simulink model "TST_Fan_DD"  (R2016b)
settings: Solver=FixedStepDiscrete  StartTime=0.0  StopTime=simTime  FixedStep=sampleTime  RelTol=1e-3
values from neighbouring files (symbols this model uses):
  testCase = 1    [initTST_Fan_DD_001.m]    (also in initTST_Fan_DD_002.m = 2)
libraries: simulink x13, UnitTest_Lib x10
settings Model: Creator=liangyunbo  LastModifiedBy=liangyunbo
settings DebuggingCC: SignalRangeChecking=error

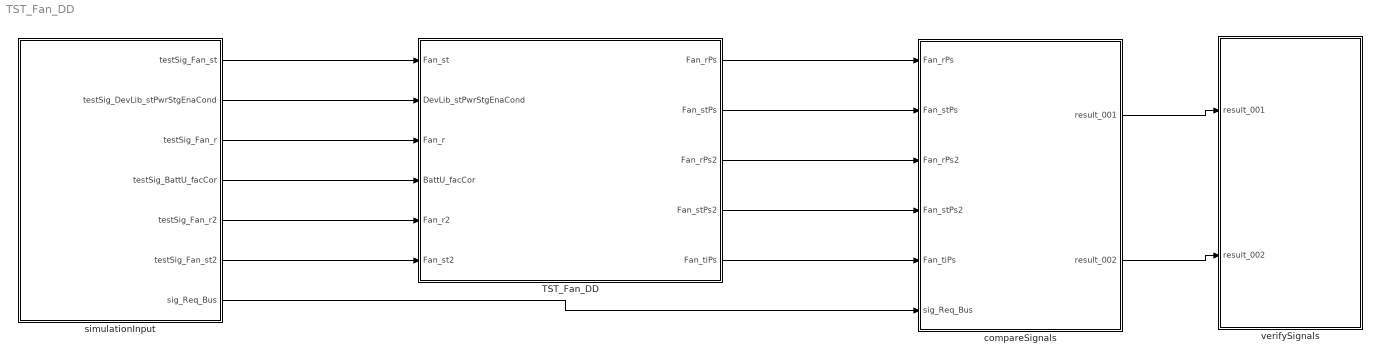
== system TST_Fan_DD ==
  TST_Fan_DD : Subsystem
  compareSignals : Subsystem
  simulationInput : Subsystem
  verifySignals : Subsystem
  wires:
  simulationInput/1(testSig_Fan_st) -> TST_Fan_DD/1(Fan_st)
  simulationInput/2(testSig_DevLib_stPwrStgEnaCond) -> TST_Fan_DD/2(DevLib_stPwrStgEnaCond)
  simulationInput/3(testSig_Fan_r) -> TST_Fan_DD/3(Fan_r)
  simulationInput/4(testSig_BattU_facCor) -> TST_Fan_DD/4(BattU_facCor)
  simulationInput/5(testSig_Fan_r2) -> TST_Fan_DD/5(Fan_r2)
  simulationInput/6(testSig_Fan_st2) -> TST_Fan_DD/6(Fan_st2)
  TST_Fan_DD/1(Fan_rPs) -> compareSignals/1(Fan_rPs)
  TST_Fan_DD/2(Fan_stPs) -> compareSignals/2(Fan_stPs)
  TST_Fan_DD/3(Fan_rPs2) -> compareSignals/3(Fan_rPs2)
  TST_Fan_DD/4(Fan_stPs2) -> compareSignals/4(Fan_stPs2)
  TST_Fan_DD/5(Fan_tiPs) -> compareSignals/5(Fan_tiPs)
  simulationInput/7(sig_Req_Bus) -> compareSignals/6(sig_Req_Bus)
  compareSignals/1(result_001) -> verifySignals/1(result_001)
  compareSignals/2(result_002) -> verifySignals/2(result_002)

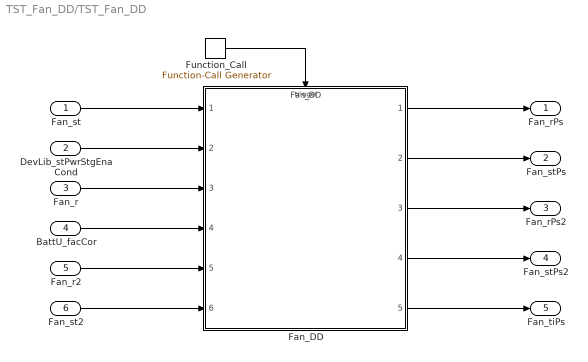
== system TST_Fan_DD/TST_Fan_DD ==
  Fan_st : Inport
  DevLib_stPwrStgEnaCond : Inport  Port=2
  Fan_r : Inport  Port=3
  BattU_facCor : Inport  Port=4
  Fan_r2 : Inport  Port=5
  Fan_st2 : Inport  Port=6
  Fan_DD : ModelReference  ModelNameDialog=Fan_DD  SimulationMode=Normal  ModelReferenceVersion=1.95  TriggerPortName=function  TriggerPortTriggerType=function-call  TriggerPortStatesWhenEnabling=held
  Function_Call : simulink/Ports & Subsystems/Function-Call Generator  sample_time=sampleTime  numberOfIterations=1
  Fan_rPs : Outport
  Fan_stPs : Outport  Port=2
  Fan_rPs2 : Outport  Port=3
  Fan_stPs2 : Outport  Port=4
  Fan_tiPs : Outport  Port=5
  wires:
  Function_Call/1 -> Fan_DD/Trigger
  Fan_st/1 -> Fan_DD/1
  DevLib_stPwrStgEnaCond/1 -> Fan_DD/2
  Fan_r/1 -> Fan_DD/3
  BattU_facCor/1 -> Fan_DD/4
  Fan_r2/1 -> Fan_DD/5
  Fan_st2/1 -> Fan_DD/6
  Fan_DD/1 -> Fan_rPs/1
  Fan_DD/2 -> Fan_stPs/1
  Fan_DD/3 -> Fan_rPs2/1
  Fan_DD/4 -> Fan_stPs2/1
  Fan_DD/5 -> Fan_tiPs/1

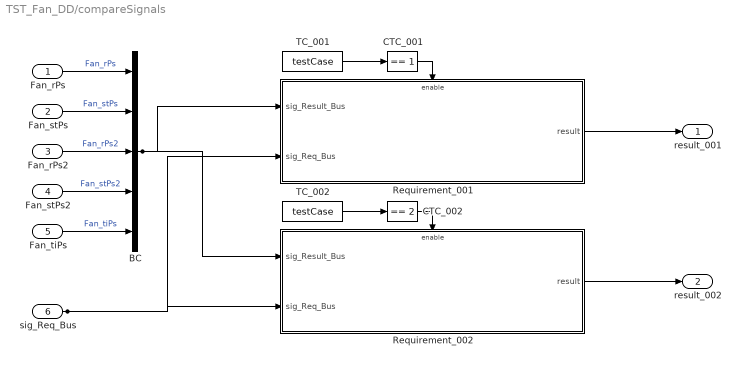
== system TST_Fan_DD/compareSignals ==
  Fan_rPs : Inport
  Fan_stPs : Inport  Port=2
  Fan_rPs2 : Inport  Port=3
  Fan_stPs2 : Inport  Port=4
  Fan_tiPs : Inport  Port=5
  sig_Req_Bus : Inport  Port=6
  BC : BusCreator  Inputs=5
  CTC_001 : simulink/Logic and Bit Operations/Compare To Constant  relop===  const=1  OutDataTypeStr=boolean
  CTC_002 : simulink/Logic and Bit Operations/Compare To Constant  relop===  const=2  OutDataTypeStr=boolean
  Requirement_001 : Subsystem
  Requirement_002 : Subsystem
  TC_001 : Constant  Value=testCase
  TC_002 : Constant  Value=testCase
  result_001 : Outport
  result_002 : Outport  Port=2
  wires:
  Fan_rPs/1 -> BC/1  "Fan_rPs"
  Fan_stPs/1 -> BC/2  "Fan_stPs"
  Fan_rPs2/1 -> BC/3  "Fan_rPs2"
  Fan_stPs2/1 -> BC/4  "Fan_stPs2"
  Fan_tiPs/1 -> BC/5  "Fan_tiPs"
  TC_001/1 -> CTC_001/1
  CTC_001/1 -> Requirement_001/Enable
  sig_Req_Bus/1 -> Requirement_001/2(sig_Req_Bus), Requirement_002/2(sig_Req_Bus)
  BC/1 -> Requirement_001/1(sig_Result_Bus), Requirement_002/1(sig_Result_Bus)
  Requirement_001/1(result) -> result_001/1
  TC_002/1 -> CTC_002/1
  CTC_002/1 -> Requirement_002/Enable
  Requirement_002/1(result) -> result_002/1

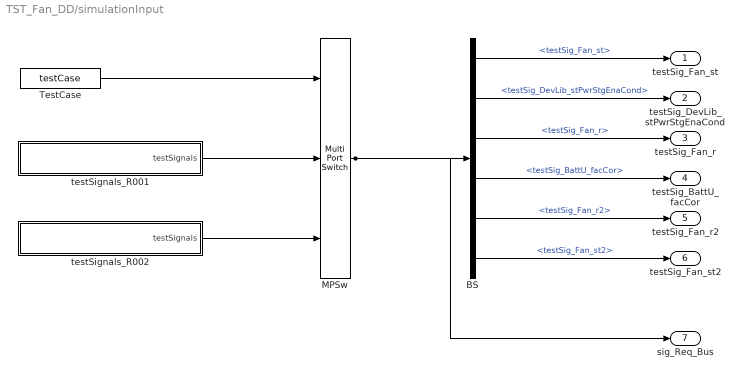
== system TST_Fan_DD/simulationInput ==
  BS : BusSelector  OutputSignals=testSig_Fan_st,testSig_DevLib_stPwrStgEnaCond,testSig_Fan_r,testSig_BattU_facCor,testSig_Fan_r2,testSig_Fan_st2
  MPSw : MultiPortSwitch  Inputs=2  SaturateOnIntegerOverflow=on  InputSameDT=on
  TestCase : Constant  Value=testCase
  testSignals_R001 : Subsystem
  testSignals_R002 : Subsystem
  testSig_Fan_st : Outport
  testSig_DevLib_stPwrStgEnaCond : Outport  Port=2
  testSig_Fan_r : Outport  Port=3
  testSig_BattU_facCor : Outport  Port=4
  testSig_Fan_r2 : Outport  Port=5
  testSig_Fan_st2 : Outport  Port=6
  sig_Req_Bus : Outport  Port=7
  wires:
  BS/1 -> testSig_Fan_st/1  "<testSig_Fan_st>"
  BS/2 -> testSig_DevLib_stPwrStgEnaCond/1  "<testSig_DevLib_stPwrStgEnaCond>"
  BS/3 -> testSig_Fan_r/1  "<testSig_Fan_r>"
  BS/4 -> testSig_BattU_facCor/1  "<testSig_BattU_facCor>"
  BS/5 -> testSig_Fan_r2/1  "<testSig_Fan_r2>"
  BS/6 -> testSig_Fan_st2/1  "<testSig_Fan_st2>"
  MPSw/1 -> BS/1, sig_Req_Bus/1
  TestCase/1 -> MPSw/1
  testSignals_R001/1(testSignals) -> MPSw/2
  testSignals_R002/1(testSignals) -> MPSw/3

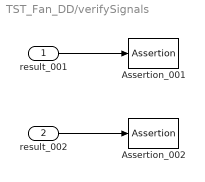
== system TST_Fan_DD/verifySignals ==
  result_001 : Inport
  result_002 : Inport  Port=2
  Assertion_001 : Assertion  Enabled=off
  Assertion_002 : Assertion  Enabled=off
  wires:
  result_001/1 -> Assertion_001/1
  result_002/1 -> Assertion_002/1

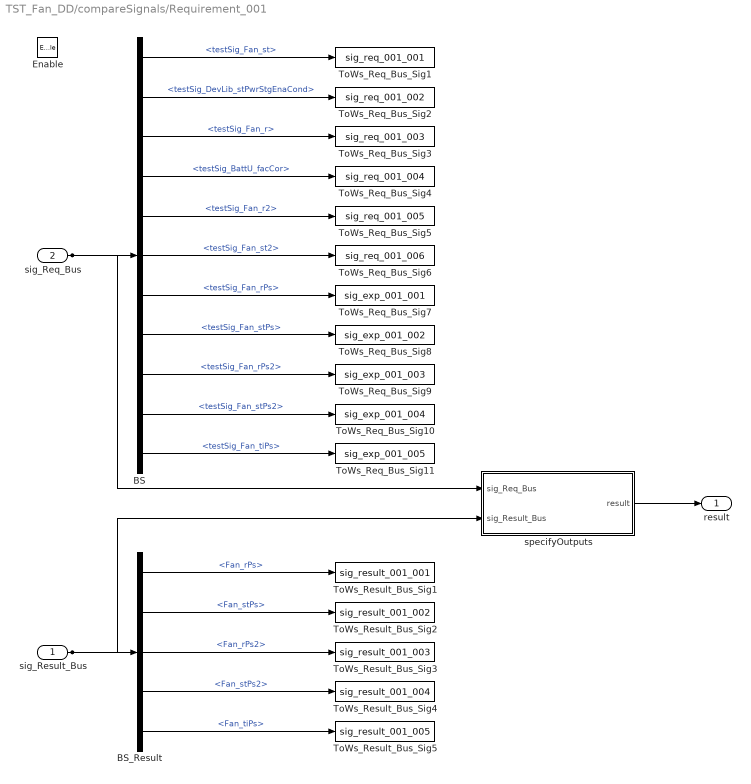
== system TST_Fan_DD/compareSignals/Requirement_001 ==
  sig_Result_Bus : Inport
  sig_Req_Bus : Inport  Port=2
  Enable : EnablePort
  BS : BusSelector  OutputSignals=testSig_Fan_st,testSig_DevLib_stPwrStgEnaCond,testSig_Fan_r,testSig_BattU_facCor,testSig_Fan_r2,testSig_Fan_st2,testSig_Fan_rPs,testSig_Fan_stPs,testSig_Fan_rPs2,testSig_Fan_stPs2,testSig_Fan_tiPs
  BS_Result : BusSelector  OutputSignals=Fan_rPs,Fan_stPs,Fan_rPs2,Fan_stPs2,Fan_tiPs
  ToWs_Req_Bus_Sig1 : ToWorkspace  VariableName=sig_req_001_001  SaveFormat=Structure With Time
  ToWs_Req_Bus_Sig10 : ToWorkspace  VariableName=sig_exp_001_004  SaveFormat=Structure With Time
  ToWs_Req_Bus_Sig11 : ToWorkspace  VariableName=sig_exp_001_005  SaveFormat=Structure With Time
  ToWs_Req_Bus_Sig2 : ToWorkspace  VariableName=sig_req_001_002  SaveFormat=Structure With Time
  ToWs_Req_Bus_Sig3 : ToWorkspace  VariableName=sig_req_001_003  SaveFormat=Structure With Time
  ToWs_Req_Bus_Sig4 : ToWorkspace  VariableName=sig_req_001_004  SaveFormat=Structure With Time
  ToWs_Req_Bus_Sig5 : ToWorkspace  VariableName=sig_req_001_005  SaveFormat=Structure With Time
  ToWs_Req_Bus_Sig6 : ToWorkspace  VariableName=sig_req_001_006  SaveFormat=Structure With Time
  ToWs_Req_Bus_Sig7 : ToWorkspace  VariableName=sig_exp_001_001  SaveFormat=Structure With Time
  ToWs_Req_Bus_Sig8 : ToWorkspace  VariableName=sig_exp_001_002  SaveFormat=Structure With Time
  ToWs_Req_Bus_Sig9 : ToWorkspace  VariableName=sig_exp_001_003  SaveFormat=Structure With Time
  ToWs_Result_Bus_Sig1 : ToWorkspace  VariableName=sig_result_001_001  SaveFormat=Structure With Time
  ToWs_Result_Bus_Sig2 : ToWorkspace  VariableName=sig_result_001_002  SaveFormat=Structure With Time
  ToWs_Result_Bus_Sig3 : ToWorkspace  VariableName=sig_result_001_003  SaveFormat=Structure With Time
  ToWs_Result_Bus_Sig4 : ToWorkspace  VariableName=sig_result_001_004  SaveFormat=Structure With Time
  ToWs_Result_Bus_Sig5 : ToWorkspace  VariableName=sig_result_001_005  SaveFormat=Structure With Time
  specifyOutputs : Subsystem
  result : Outport
  wires:
  sig_Req_Bus/1 -> BS/1, specifyOutputs/1(sig_Req_Bus)
  BS/1 -> ToWs_Req_Bus_Sig1/1  "<testSig_Fan_st>"
  BS/2 -> ToWs_Req_Bus_Sig2/1  "<testSig_DevLib_stPwrStgEnaCond>"
  BS/3 -> ToWs_Req_Bus_Sig3/1  "<testSig_Fan_r>"
  BS/4 -> ToWs_Req_Bus_Sig4/1  "<testSig_BattU_facCor>"
  BS/5 -> ToWs_Req_Bus_Sig5/1  "<testSig_Fan_r2>"
  BS/6 -> ToWs_Req_Bus_Sig6/1  "<testSig_Fan_st2>"
  BS/7 -> ToWs_Req_Bus_Sig7/1  "<testSig_Fan_rPs>"
  BS/8 -> ToWs_Req_Bus_Sig8/1  "<testSig_Fan_stPs>"
  BS/9 -> ToWs_Req_Bus_Sig9/1  "<testSig_Fan_rPs2>"
  BS/10 -> ToWs_Req_Bus_Sig10/1  "<testSig_Fan_stPs2>"
  BS/11 -> ToWs_Req_Bus_Sig11/1  "<testSig_Fan_tiPs>"
  sig_Result_Bus/1 -> BS_Result/1, specifyOutputs/2(sig_Result_Bus)
  BS_Result/1 -> ToWs_Result_Bus_Sig1/1  "<Fan_rPs>"
  BS_Result/2 -> ToWs_Result_Bus_Sig2/1  "<Fan_stPs>"
  BS_Result/3 -> ToWs_Result_Bus_Sig3/1  "<Fan_rPs2>"
  BS_Result/4 -> ToWs_Result_Bus_Sig4/1  "<Fan_stPs2>"
  BS_Result/5 -> ToWs_Result_Bus_Sig5/1  "<Fan_tiPs>"
  specifyOutputs/1(result) -> result/1

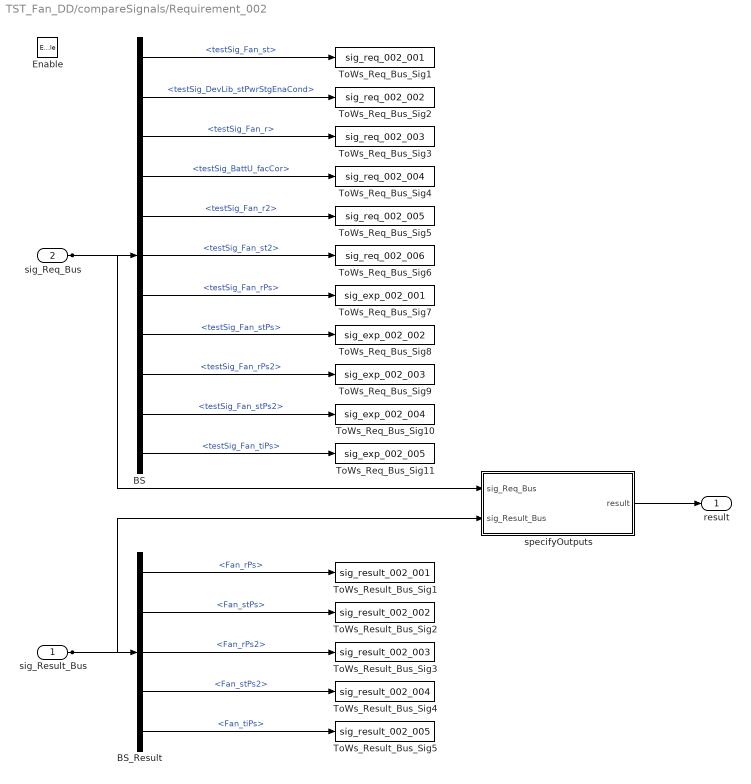
== system TST_Fan_DD/compareSignals/Requirement_002 ==
  sig_Result_Bus : Inport
  sig_Req_Bus : Inport  Port=2
  Enable : EnablePort
  BS : BusSelector  OutputSignals=testSig_Fan_st,testSig_DevLib_stPwrStgEnaCond,testSig_Fan_r,testSig_BattU_facCor,testSig_Fan_r2,testSig_Fan_st2,testSig_Fan_rPs,testSig_Fan_stPs,testSig_Fan_rPs2,testSig_Fan_stPs2,testSig_Fan_tiPs
  BS_Result : BusSelector  OutputSignals=Fan_rPs,Fan_stPs,Fan_rPs2,Fan_stPs2,Fan_tiPs
  ToWs_Req_Bus_Sig1 : ToWorkspace  VariableName=sig_req_002_001  SaveFormat=Structure With Time
  ToWs_Req_Bus_Sig10 : ToWorkspace  VariableName=sig_exp_002_004  SaveFormat=Structure With Time
  ToWs_Req_Bus_Sig11 : ToWorkspace  VariableName=sig_exp_002_005  SaveFormat=Structure With Time
  ToWs_Req_Bus_Sig2 : ToWorkspace  VariableName=sig_req_002_002  SaveFormat=Structure With Time
  ToWs_Req_Bus_Sig3 : ToWorkspace  VariableName=sig_req_002_003  SaveFormat=Structure With Time
  ToWs_Req_Bus_Sig4 : ToWorkspace  VariableName=sig_req_002_004  SaveFormat=Structure With Time
  ToWs_Req_Bus_Sig5 : ToWorkspace  VariableName=sig_req_002_005  SaveFormat=Structure With Time
  ToWs_Req_Bus_Sig6 : ToWorkspace  VariableName=sig_req_002_006  SaveFormat=Structure With Time
  ToWs_Req_Bus_Sig7 : ToWorkspace  VariableName=sig_exp_002_001  SaveFormat=Structure With Time
  ToWs_Req_Bus_Sig8 : ToWorkspace  VariableName=sig_exp_002_002  SaveFormat=Structure With Time
  ToWs_Req_Bus_Sig9 : ToWorkspace  VariableName=sig_exp_002_003  SaveFormat=Structure With Time
  ToWs_Result_Bus_Sig1 : ToWorkspace  VariableName=sig_result_002_001  SaveFormat=Structure With Time
  ToWs_Result_Bus_Sig2 : ToWorkspace  VariableName=sig_result_002_002  SaveFormat=Structure With Time
  ToWs_Result_Bus_Sig3 : ToWorkspace  VariableName=sig_result_002_003  SaveFormat=Structure With Time
  ToWs_Result_Bus_Sig4 : ToWorkspace  VariableName=sig_result_002_004  SaveFormat=Structure With Time
  ToWs_Result_Bus_Sig5 : ToWorkspace  VariableName=sig_result_002_005  SaveFormat=Structure With Time
  specifyOutputs : Subsystem
  result : Outport
  wires:
  sig_Req_Bus/1 -> BS/1, specifyOutputs/1(sig_Req_Bus)
  BS/1 -> ToWs_Req_Bus_Sig1/1  "<testSig_Fan_st>"
  BS/2 -> ToWs_Req_Bus_Sig2/1  "<testSig_DevLib_stPwrStgEnaCond>"
  BS/3 -> ToWs_Req_Bus_Sig3/1  "<testSig_Fan_r>"
  BS/4 -> ToWs_Req_Bus_Sig4/1  "<testSig_BattU_facCor>"
  BS/5 -> ToWs_Req_Bus_Sig5/1  "<testSig_Fan_r2>"
  BS/6 -> ToWs_Req_Bus_Sig6/1  "<testSig_Fan_st2>"
  BS/7 -> ToWs_Req_Bus_Sig7/1  "<testSig_Fan_rPs>"
  BS/8 -> ToWs_Req_Bus_Sig8/1  "<testSig_Fan_stPs>"
  BS/9 -> ToWs_Req_Bus_Sig9/1  "<testSig_Fan_rPs2>"
  BS/10 -> ToWs_Req_Bus_Sig10/1  "<testSig_Fan_stPs2>"
  BS/11 -> ToWs_Req_Bus_Sig11/1  "<testSig_Fan_tiPs>"
  sig_Result_Bus/1 -> BS_Result/1, specifyOutputs/2(sig_Result_Bus)
  BS_Result/1 -> ToWs_Result_Bus_Sig1/1  "<Fan_rPs>"
  BS_Result/2 -> ToWs_Result_Bus_Sig2/1  "<Fan_stPs>"
  BS_Result/3 -> ToWs_Result_Bus_Sig3/1  "<Fan_rPs2>"
  BS_Result/4 -> ToWs_Result_Bus_Sig4/1  "<Fan_stPs2>"
  BS_Result/5 -> ToWs_Result_Bus_Sig5/1  "<Fan_tiPs>"
  specifyOutputs/1(result) -> result/1

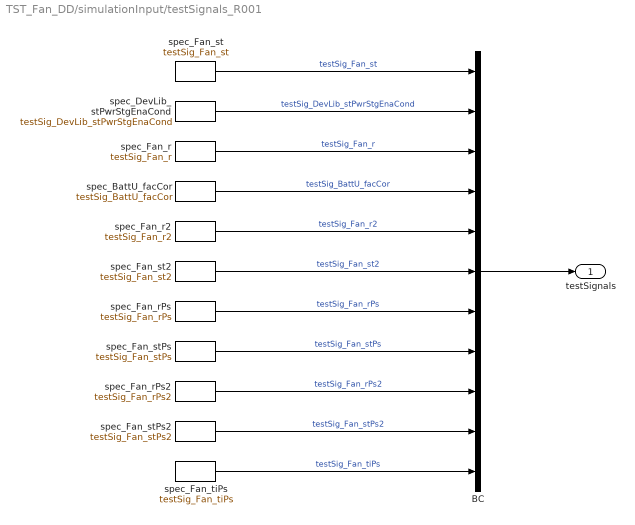
== system TST_Fan_DD/simulationInput/testSignals_R001 ==
  BC : BusCreator  Inputs=11
  spec_BattU_facCor : FromWorkspace  VariableName=testSig_BattU_facCor  Interpolate=off  OutputAfterFinalValue=Holding final value
  spec_DevLib_stPwrStgEnaCond : FromWorkspace  VariableName=testSig_DevLib_stPwrStgEnaCond  Interpolate=off  OutputAfterFinalValue=Holding final value
  spec_Fan_r : FromWorkspace  VariableName=testSig_Fan_r  Interpolate=off  OutputAfterFinalValue=Holding final value
  spec_Fan_r2 : FromWorkspace  VariableName=testSig_Fan_r2  Interpolate=off  OutputAfterFinalValue=Holding final value
  spec_Fan_rPs : FromWorkspace  VariableName=testSig_Fan_rPs  Interpolate=off  OutputAfterFinalValue=Holding final value
  spec_Fan_rPs2 : FromWorkspace  VariableName=testSig_Fan_rPs2  Interpolate=off  OutputAfterFinalValue=Holding final value
  spec_Fan_st : FromWorkspace  VariableName=testSig_Fan_st  Interpolate=off  OutputAfterFinalValue=Holding final value
  spec_Fan_st2 : FromWorkspace  VariableName=testSig_Fan_st2  Interpolate=off  OutputAfterFinalValue=Holding final value
  spec_Fan_stPs : FromWorkspace  VariableName=testSig_Fan_stPs  Interpolate=off  OutputAfterFinalValue=Holding final value
  spec_Fan_stPs2 : FromWorkspace  VariableName=testSig_Fan_stPs2  Interpolate=off  OutputAfterFinalValue=Holding final value
  spec_Fan_tiPs : FromWorkspace  VariableName=testSig_Fan_tiPs  Interpolate=off  OutputAfterFinalValue=Holding final value
  testSignals : Outport
  wires:
  BC/1 -> testSignals/1
  spec_Fan_st/1 -> BC/1  "testSig_Fan_st"
  spec_DevLib_stPwrStgEnaCond/1 -> BC/2  "testSig_DevLib_stPwrStgEnaCond"
  spec_Fan_r/1 -> BC/3  "testSig_Fan_r"
  spec_BattU_facCor/1 -> BC/4  "testSig_BattU_facCor"
  spec_Fan_r2/1 -> BC/5  "testSig_Fan_r2"
  spec_Fan_st2/1 -> BC/6  "testSig_Fan_st2"
  spec_Fan_rPs/1 -> BC/7  "testSig_Fan_rPs"
  spec_Fan_stPs/1 -> BC/8  "testSig_Fan_stPs"
  spec_Fan_rPs2/1 -> BC/9  "testSig_Fan_rPs2"
  spec_Fan_stPs2/1 -> BC/10  "testSig_Fan_stPs2"
  spec_Fan_tiPs/1 -> BC/11  "testSig_Fan_tiPs"

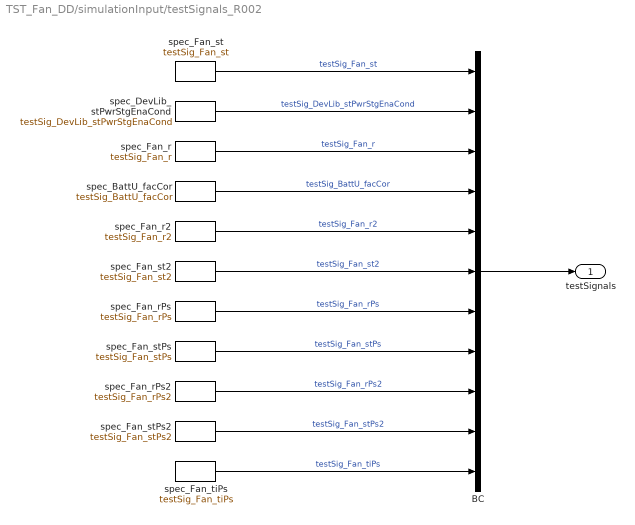
== system TST_Fan_DD/simulationInput/testSignals_R002 ==
  BC : BusCreator  Inputs=11
  spec_BattU_facCor : FromWorkspace  VariableName=testSig_BattU_facCor  Interpolate=off  OutputAfterFinalValue=Holding final value
  spec_DevLib_stPwrStgEnaCond : FromWorkspace  VariableName=testSig_DevLib_stPwrStgEnaCond  Interpolate=off  OutputAfterFinalValue=Holding final value
  spec_Fan_r : FromWorkspace  VariableName=testSig_Fan_r  Interpolate=off  OutputAfterFinalValue=Holding final value
  spec_Fan_r2 : FromWorkspace  VariableName=testSig_Fan_r2  Interpolate=off  OutputAfterFinalValue=Holding final value
  spec_Fan_rPs : FromWorkspace  VariableName=testSig_Fan_rPs  Interpolate=off  OutputAfterFinalValue=Holding final value
  spec_Fan_rPs2 : FromWorkspace  VariableName=testSig_Fan_rPs2  Interpolate=off  OutputAfterFinalValue=Holding final value
  spec_Fan_st : FromWorkspace  VariableName=testSig_Fan_st  Interpolate=off  OutputAfterFinalValue=Holding final value
  spec_Fan_st2 : FromWorkspace  VariableName=testSig_Fan_st2  Interpolate=off  OutputAfterFinalValue=Holding final value
  spec_Fan_stPs : FromWorkspace  VariableName=testSig_Fan_stPs  Interpolate=off  OutputAfterFinalValue=Holding final value
  spec_Fan_stPs2 : FromWorkspace  VariableName=testSig_Fan_stPs2  Interpolate=off  OutputAfterFinalValue=Holding final value
  spec_Fan_tiPs : FromWorkspace  VariableName=testSig_Fan_tiPs  Interpolate=off  OutputAfterFinalValue=Holding final value
  testSignals : Outport
  wires:
  BC/1 -> testSignals/1
  spec_Fan_st/1 -> BC/1  "testSig_Fan_st"
  spec_DevLib_stPwrStgEnaCond/1 -> BC/2  "testSig_DevLib_stPwrStgEnaCond"
  spec_Fan_r/1 -> BC/3  "testSig_Fan_r"
  spec_BattU_facCor/1 -> BC/4  "testSig_BattU_facCor"
  spec_Fan_r2/1 -> BC/5  "testSig_Fan_r2"
  spec_Fan_st2/1 -> BC/6  "testSig_Fan_st2"
  spec_Fan_rPs/1 -> BC/7  "testSig_Fan_rPs"
  spec_Fan_stPs/1 -> BC/8  "testSig_Fan_stPs"
  spec_Fan_rPs2/1 -> BC/9  "testSig_Fan_rPs2"
  spec_Fan_stPs2/1 -> BC/10  "testSig_Fan_stPs2"
  spec_Fan_tiPs/1 -> BC/11  "testSig_Fan_tiPs"

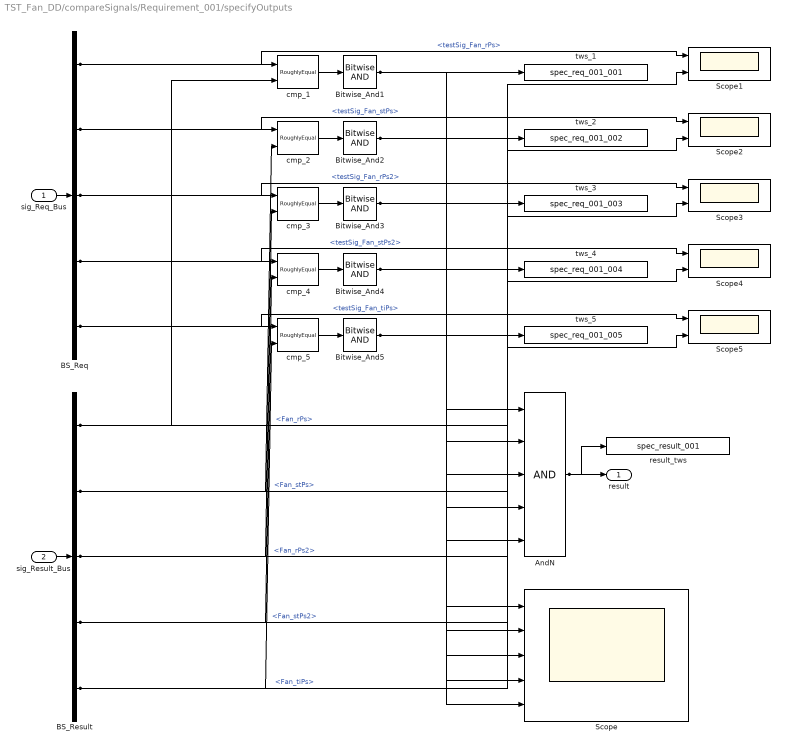
== system TST_Fan_DD/compareSignals/Requirement_001/specifyOutputs ==
  sig_Req_Bus : Inport
  sig_Result_Bus : Inport  Port=2
  AndN : Logic  Inputs=5
  BS_Req : BusSelector  OutputSignals=testSig_Fan_rPs,testSig_Fan_stPs,testSig_Fan_rPs2,testSig_Fan_stPs2,testSig_Fan_tiPs
  BS_Result : BusSelector  OutputSignals=Fan_rPs,Fan_stPs,Fan_rPs2,Fan_stPs2,Fan_tiPs
  Bitwise_And{1..5} (5 alike) : simulink/Logic and Bit Operations/Bitwise Operator  logicop=AND  UseBitMask=off  BitMask=bin2dec('11011001')  BitMaskRealWorld=Stored Integer
  Scope : Scope  NumInputPorts=5
  Scope{1..5} (5 alike) : Scope  NumInputPorts=2
  cmp_{1..5} (5 alike) : UnitTest_Lib/RoughlyEqual  slope=0.1
  result_tws : ToWorkspace  VariableName=spec_result_001
  tws_1 : ToWorkspace  VariableName=spec_req_001_001
  tws_2 : ToWorkspace  VariableName=spec_req_001_002
  tws_3 : ToWorkspace  VariableName=spec_req_001_003
  tws_4 : ToWorkspace  VariableName=spec_req_001_004
  tws_5 : ToWorkspace  VariableName=spec_req_001_005
  result : Outport
  wires:
  sig_Req_Bus/1 -> BS_Req/1
  sig_Result_Bus/1 -> BS_Result/1
  AndN/1 -> result/1, result_tws/1
  BS_Req/1 -> cmp_1/1, Scope1/1  "<testSig_Fan_rPs>"
  BS_Result/1 -> cmp_1/2, Scope1/2  "<Fan_rPs>"
  cmp_1/1 -> Bitwise_And1/1
  Bitwise_And1/1 -> tws_1/1, AndN/1, Scope/1
  BS_Req/2 -> cmp_2/1, Scope2/1  "<testSig_Fan_stPs>"
  BS_Result/2 -> cmp_2/2, Scope2/2  "<Fan_stPs>"
  cmp_2/1 -> Bitwise_And2/1
  Bitwise_And2/1 -> tws_2/1, AndN/2, Scope/2
  BS_Req/3 -> cmp_3/1, Scope3/1  "<testSig_Fan_rPs2>"
  BS_Result/3 -> cmp_3/2, Scope3/2  "<Fan_rPs2>"
  cmp_3/1 -> Bitwise_And3/1
  Bitwise_And3/1 -> tws_3/1, AndN/3, Scope/3
  BS_Req/4 -> cmp_4/1, Scope4/1  "<testSig_Fan_stPs2>"
  BS_Result/4 -> cmp_4/2, Scope4/2  "<Fan_stPs2>"
  cmp_4/1 -> Bitwise_And4/1
  Bitwise_And4/1 -> tws_4/1, AndN/4, Scope/4
  BS_Req/5 -> cmp_5/1, Scope5/1  "<testSig_Fan_tiPs>"
  BS_Result/5 -> cmp_5/2, Scope5/2  "<Fan_tiPs>"
  cmp_5/1 -> Bitwise_And5/1
  Bitwise_And5/1 -> tws_5/1, AndN/5, Scope/5

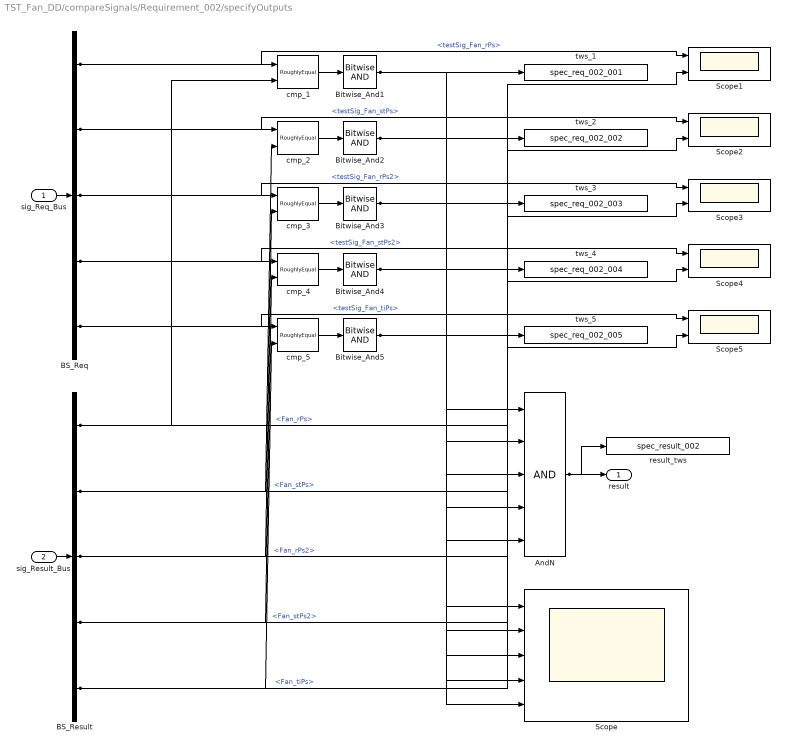
== system TST_Fan_DD/compareSignals/Requirement_002/specifyOutputs ==
  sig_Req_Bus : Inport
  sig_Result_Bus : Inport  Port=2
  AndN : Logic  Inputs=5
  BS_Req : BusSelector  OutputSignals=testSig_Fan_rPs,testSig_Fan_stPs,testSig_Fan_rPs2,testSig_Fan_stPs2,testSig_Fan_tiPs
  BS_Result : BusSelector  OutputSignals=Fan_rPs,Fan_stPs,Fan_rPs2,Fan_stPs2,Fan_tiPs
  Bitwise_And{1..5} (5 alike) : simulink/Logic and Bit Operations/Bitwise Operator  logicop=AND  UseBitMask=off  BitMask=bin2dec('11011001')  BitMaskRealWorld=Stored Integer
  Scope : Scope  NumInputPorts=5
  Scope{1..5} (5 alike) : Scope  NumInputPorts=2
  cmp_{1..5} (5 alike) : UnitTest_Lib/RoughlyEqual  slope=0.1
  result_tws : ToWorkspace  VariableName=spec_result_002
  tws_1 : ToWorkspace  VariableName=spec_req_002_001
  tws_2 : ToWorkspace  VariableName=spec_req_002_002
  tws_3 : ToWorkspace  VariableName=spec_req_002_003
  tws_4 : ToWorkspace  VariableName=spec_req_002_004
  tws_5 : ToWorkspace  VariableName=spec_req_002_005
  result : Outport
  wires:
  sig_Req_Bus/1 -> BS_Req/1
  sig_Result_Bus/1 -> BS_Result/1
  AndN/1 -> result/1, result_tws/1
  BS_Req/1 -> cmp_1/1, Scope1/1  "<testSig_Fan_rPs>"
  BS_Result/1 -> cmp_1/2, Scope1/2  "<Fan_rPs>"
  cmp_1/1 -> Bitwise_And1/1
  Bitwise_And1/1 -> tws_1/1, AndN/1, Scope/1
  BS_Req/2 -> cmp_2/1, Scope2/1  "<testSig_Fan_stPs>"
  BS_Result/2 -> cmp_2/2, Scope2/2  "<Fan_stPs>"
  cmp_2/1 -> Bitwise_And2/1
  Bitwise_And2/1 -> tws_2/1, AndN/2, Scope/2
  BS_Req/3 -> cmp_3/1, Scope3/1  "<testSig_Fan_rPs2>"
  BS_Result/3 -> cmp_3/2, Scope3/2  "<Fan_rPs2>"
  cmp_3/1 -> Bitwise_And3/1
  Bitwise_And3/1 -> tws_3/1, AndN/3, Scope/3
  BS_Req/4 -> cmp_4/1, Scope4/1  "<testSig_Fan_stPs2>"
  BS_Result/4 -> cmp_4/2, Scope4/2  "<Fan_stPs2>"
  cmp_4/1 -> Bitwise_And4/1
  Bitwise_And4/1 -> tws_4/1, AndN/4, Scope/4
  BS_Req/5 -> cmp_5/1, Scope5/1  "<testSig_Fan_tiPs>"
  BS_Result/5 -> cmp_5/2, Scope5/2  "<Fan_tiPs>"
  cmp_5/1 -> Bitwise_And5/1
  Bitwise_And5/1 -> tws_5/1, AndN/5, Scope/5
